simulink model "pwaSys_obs_model"  (Simulink 8.6)
settings: Solver=ode45  StartTime=0.0  StopTime=sim_T  RelTol=1e-3
InitFcn:
  | load simulink.mat
  | setParameters
StartFcn:
  | load simulink.mat
  | setParameters
  | clear res_X res_U res_Y res_P res_D
  | clear res_Xest res_Dest res_Yest
StopFcn:
  | plotScope
undefined symbols (not defined in the file or in its folder): sim_nx, sim_ny, sim_x0
undefined symbols (not defined in the file): sim_A, sim_Aobs, sim_B, sim_Bobs, sim_C, sim_Cobs, sim_D, sim_d0obs, sim_Dobs, sim_H, sim_Hobs, sim_K, sim_Kobs, sim_TsObs, sim_x0obs
settings Model: Creator=alberto  LastModifiedBy=root
settings DataIOCC: SignalLoggingSaveFormat=Dataset
settings OptimizationCC: ExpressionDepthLimit=128
settings DebuggingCC: UnderspecifiedInitializationDetection=Simplified  MergeDetectMultiDrivingBlocksExec=error  FcnCallInpInsideContextMsg=EnableAllAsError  StateNameClashWarn=none
settings GRTTargetCC: CombineOutputUpdateFcns=on  GRTInterface=off
settings ConfigComp: CovSFcnEnable=off

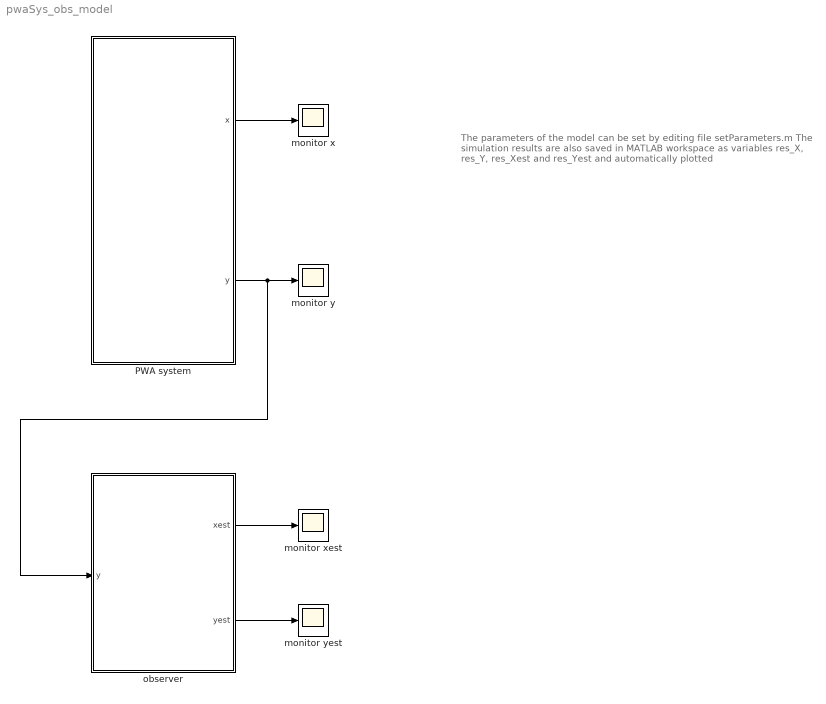
== system pwaSys_obs_model ==
  note: The parameters of the model can be set by editing file setParameters.m
      |
      | The simulation results are also saved in MATLAB workspace as variables
      | res_X, res_Y, res_Xest and res_Yest and automatically plotted
  PWA system : Subsystem
  monitor x : Scope
  monitor xest : Scope
  monitor y : Scope
  monitor yest : Scope
  observer : Subsystem
  wires:
  PWA system/1(x) -> monitor x/1
  PWA system/2(y) -> observer/1(y), monitor y/1
  observer/1(xest) -> monitor xest/1
  observer/2(yest) -> monitor yest/1

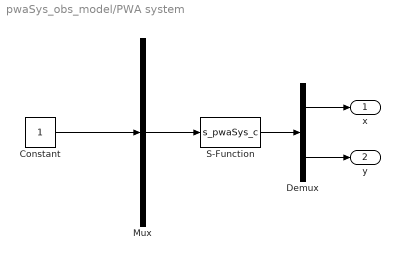
== system pwaSys_obs_model/PWA system ==
  Constant : Constant
  Demux : Demux  Outputs=[sim_nx sim_ny]
  Mux : Mux  Inputs=1
  S-Function : S-Function  FunctionName=s_pwaSys_c  Parameters=A,B,C,D,H,K,sim_x0  SFunctionDeploymentMode=off  EnableBusSupport=off  mask{A=sim_A, B=sim_B, C=sim_C, D=sim_D, H=sim_H, K=sim_K, sim_x0=sim_x0}
      mask prompts: sim_x0 "Initial condition"
      mask DialogControl DescTextVar Prompt: continuous time PWA system
  x : Outport
  y : Outport  Port=2
  wires:
  Mux/1 -> S-Function/1
  S-Function/1 -> Demux/1
  Demux/1 -> x/1
  Demux/2 -> y/1
  Constant/1 -> Mux/1

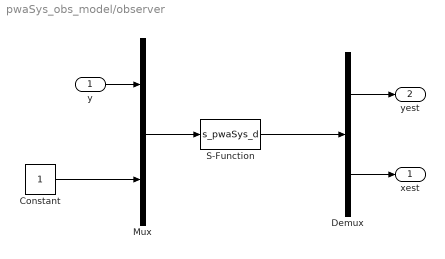
== system pwaSys_obs_model/observer ==
  y : Inport
  Constant : Constant
  Demux : Demux  Outputs=[sim_ny sim_nx]
  Mux : Mux  Inputs=2
  S-Function : S-Function  FunctionName=s_pwaSys_d  Parameters=A,B,C,D,H,K,sim_x0,Ts  SFunctionDeploymentMode=off  EnableBusSupport=off  mask{A=sim_Aobs, B=sim_Bobs, C=sim_Cobs, D=sim_Dobs, H=sim_Hobs, K=sim_Kobs, sim_x0=[sim_x0obs;sim_d0obs], Ts=sim_TsObs}
      mask prompts: sim_x0 "Initial condition"; Ts "Sample time"
      mask DialogControl DescTextVar Prompt: continuous time PWA system
  xest : Outport
  yest : Outport  Port=2
  wires:
  Mux/1 -> S-Function/1
  S-Function/1 -> Demux/1
  Constant/1 -> Mux/2
  y/1 -> Mux/1
  Demux/1 -> yest/1
  Demux/2 -> xest/1
